simulink model "FOC_Controller"  (R2021a)
settings: Solver=FixedStepDiscrete  StartTime=0.0  StopTime=inf  FixedStep=4e-6  RelTol=1e-3
values from neighbouring files (symbols this model uses):
  FOC_bManualVdVq_C = Simulink.Parameter    [modeldata.m]
  FOC_iIdSP_C = Simulink.Parameter    [modeldata.m]
  FOC_kiPID_C = Simulink.Parameter    [modeldata.m]
  FOC_kpPID_C = Simulink.Parameter    [modeldata.m]
  FOC_uBusVoltage_C = Simulink.Parameter    [modeldata.m]
  FOC_uFindPosVd_C = Simulink.Parameter    [modeldata.m]
  FOC_uManualVd_C = Simulink.Parameter    [modeldata.m]
  FOC_uManualVq_C = Simulink.Parameter    [modeldata.m]
  Motor_bFindPosEnable_C = Simulink.Parameter    [modeldata.m]
  Motor_facTrq2Current_C = Simulink.Parameter    [modeldata.m]
  Motor_swtMode_C = Simulink.Parameter    [modeldata.m]
  Motor_tiFindPos_C = Simulink.Parameter    [modeldata.m]
  Motor_trqTorqueSetPoint_C = Simulink.Parameter    [modeldata.m]
  Position_degSetPoint_C = Simulink.Parameter    [modeldata.m]
  Position_kiPID_C = Simulink.Parameter    [modeldata.m]
  Position_kpPID_C = Simulink.Parameter    [modeldata.m]
  Position_nPIDMax_C = Simulink.Parameter    [modeldata.m]
  Speed_iPIDMax_C = Simulink.Parameter    [modeldata.m]
  Speed_kiPID_C = Simulink.Parameter    [modeldata.m]
  Speed_kpPID_C = Simulink.Parameter    [modeldata.m]
  Speed_nSetPoint_C = Simulink.Parameter    [modeldata.m]
  Speed_tiFilter_C = Simulink.Parameter    [modeldata.m]
libraries: simulink x11
(part 1 of 2)
settings Model: Creator=Administrator  LastModifiedBy=Administrator
settings SolverCC: AlgebraicLoopSolver=TrustRegion
settings DataIOCC: LimitDataPoints=on  ReturnWorkspaceOutputs=off
settings OptimizationCC: BlockReduction=off  DefaultParameterBehavior=Inlined  DefaultUnderspecifiedDataType=single  LifeSpan=1  EfficientTunableParamExpr=on
settings DebuggingCC: SignalInfNanChecking=warning  UnderspecifiedInitializationDetection=Classic  MergeDetectMultiDrivingBlocksExec=none  MultiTaskCondExecSysMsg=warning  MultiTaskRateTransMsg=warning  ParameterPrecisionLossMsg=none  SFUnexpectedBacktrackingDiag=warning  SFNoUnconditionalDefaultTransitionDiag=warning  SFExecutionAtInitializationDiag=none  SFMachineParentedDataDiag=warning  ArithmeticOperatorsInVariantConditions=warning
settings HardwareCC: ProdBitPerPointer=32  ProdBitPerSizeT=32  ProdBitPerPtrDiffT=32  ProdLargestAtomicInteger=Long  ProdLargestAtomicFloat=Double  ProdWordSize=32  ProdHWDeviceType=ARM Compatible->ARM Cortex
settings ModelReferenceCC: PropagateSignalLabelsOutOfModel=off
settings SFSimCC: SimUseLocalCustomCode=off  MATLABDynamicMemAlloc=off  CustomCodeUndefinedFunction=UseInterfaceOnly
settings RTWCC: SystemTargetFile=ert.tlc  GenCodeOnly=on  PackageName=AccPedal  TemplateMakefile=ert_default_tmf  GenerateReport=on  RTWVerbose=off  RTWUseLocalCustomCode=off  IncludeHyperlinkInReport=on  LaunchReport=on
settings CodeAppCC: IgnoreCustomStorageClasses=off  MaxIdLength=63  StateflowObjectComments=on
settings ERTTargetCC: TargetLangStandard=C99 (ISO)  MultiwordLength=2048  SupportNonFinite=off  ExtModeTransport=1  ExtModeMexFile=ext_serial_win32_comm  ERTCustomFileTemplate=example_file_process.tlc  ConvertIfToSwitch=off  SuppressUnreachableDefaultCases=off
settings ConfigComp: CovMetricSettings=dw  CovSaveCumulativeToWorkspaceVar=on  CovSaveSingleToWorkspaceVar=on  CovExternalEMLEnable=off  DVMaxProcessTime=600  DVMaxTestCaseSteps=500  DVTestSuiteOptimization=CombinedObjectives (Nonlinear Extended)  DVSaveReport=on
settings SimscapeCC: SimscapeNormalizeSystem=off

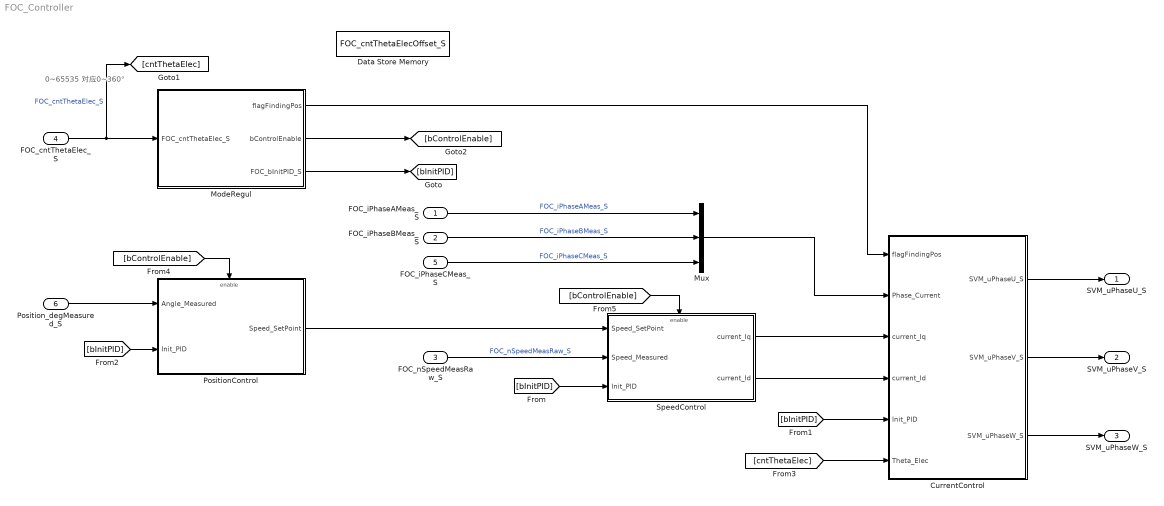
== system FOC_Controller ==
  note: 0~65535
      | 对应0~360°
  FOC_iPhaseAMeas_S : Inport  OutDataTypeStr=single
  FOC_iPhaseBMeas_S : Inport  Port=2  OutDataTypeStr=single
  FOC_nSpeedMeasRaw_S : Inport  Port=3
  FOC_cntThetaElec_S : Inport  Port=4
  FOC_iPhaseCMeas_S : Inport  Port=5  OutDataTypeStr=single
  Position_degMeasured_S : Inport  Port=6  OutDataTypeStr=single
  CurrentControl : Subsystem  TreatAsAtomicUnit=on  SystemSampleTime=200e-6  RTWFcnName=CurrentControl_Co  RTWFileName=CurrentControl
      settings: RTWSystemCode=Nonreusable function  RTWFcnNameOpts=User specified  RTWFileNameOpts=User specified
      settings: AttributesFormatString=|
      | ---------------------------------------
      | SampeTime = %<SystemSampleTime>
  Data Store Memory : DataStoreMemory  DataStoreName=FOC_cntThetaElecOffset_S  ReadBeforeWriteMsg=warning  WriteAfterWriteMsg=warning  WriteAfterReadMsg=warning  ShowAdditionalParam=off  StateMustResolveToSignalObject=on
  ModeRegul : Subsystem  TreatAsAtomicUnit=on  SystemSampleTime=0.05  RTWFcnName=ModeRegul_Co  RTWFileName=ModeRegul
      settings: RTWSystemCode=Nonreusable function  RTWFcnNameOpts=User specified  RTWFileNameOpts=User specified
      settings: AttributesFormatString=|
      | ---------------------------------------
      | SampeTime = %<SystemSampleTime>
  Mux : Mux  Inputs=3
  PositionControl : Subsystem  TreatAsAtomicUnit=on  SystemSampleTime=0.01  RTWFcnName=PositionControl_Co  RTWFileName=PositionControl
      settings: RTWSystemCode=Nonreusable function  RTWFcnNameOpts=User specified  RTWFileNameOpts=User specified
      settings: AttributesFormatString=|
      | ---------------------------------------
      | SampeTime = %<SystemSampleTime>
  SpeedControl : Subsystem  TreatAsAtomicUnit=on  SystemSampleTime=0.01  RTWFcnName=SpeedControl_Co  RTWFileName=SpeedControl
      settings: RTWSystemCode=Nonreusable function  RTWFcnNameOpts=User specified  RTWFileNameOpts=User specified
      settings: AttributesFormatString=|
      | ---------------------------------------
      | SampeTime = %<SystemSampleTime>
  SVM_uPhaseU_S : Outport  VectorParamsAs1DForOutWhenUnconnected=off
  SVM_uPhaseV_S : Outport  Port=2  VectorParamsAs1DForOutWhenUnconnected=off
  SVM_uPhaseW_S : Outport  Port=3  VectorParamsAs1DForOutWhenUnconnected=off
  wires:
  SpeedControl/1(current_Iq) -> CurrentControl/3(current_Iq)
  FOC_cntThetaElec_S/1 -> [cntThetaElec], ModeRegul/1(FOC_cntThetaElec_S)  "FOC_cntThetaElec_S"
  FOC_nSpeedMeasRaw_S/1 -> SpeedControl/2(Speed_Measured)  "FOC_nSpeedMeasRaw_S"
  Mux/1 -> CurrentControl/2(Phase_Current)
  [bInitPID] -> SpeedControl/3(Init_PID)
  FOC_iPhaseAMeas_S/1 -> Mux/1  "FOC_iPhaseAMeas_S"
  FOC_iPhaseBMeas_S/1 -> Mux/2  "FOC_iPhaseBMeas_S"
  FOC_iPhaseCMeas_S/1 -> Mux/3  "FOC_iPhaseCMeas_S"
  CurrentControl/1(SVM_uPhaseU_S) -> SVM_uPhaseU_S/1
  CurrentControl/3(SVM_uPhaseW_S) -> SVM_uPhaseW_S/1
  CurrentControl/2(SVM_uPhaseV_S) -> SVM_uPhaseV_S/1
  PositionControl/1(Speed_SetPoint) -> SpeedControl/1(Speed_SetPoint)
  [bInitPID] -> CurrentControl/5(Init_PID)
  Position_degMeasured_S/1 -> PositionControl/1(Angle_Measured)
  ModeRegul/3(FOC_bInitPID_S) -> [bInitPID]
  [bInitPID] -> PositionControl/2(Init_PID)
  [cntThetaElec] -> CurrentControl/6(Theta_Elec)
  ModeRegul/1(flagFindingPos) -> CurrentControl/1(flagFindingPos)
  ModeRegul/2(bControlEnable) -> [bControlEnable]
  [bControlEnable] -> PositionControl/Enable
  [bControlEnable] -> SpeedControl/Enable
  SpeedControl/2(current_Id) -> CurrentControl/4(current_Id)

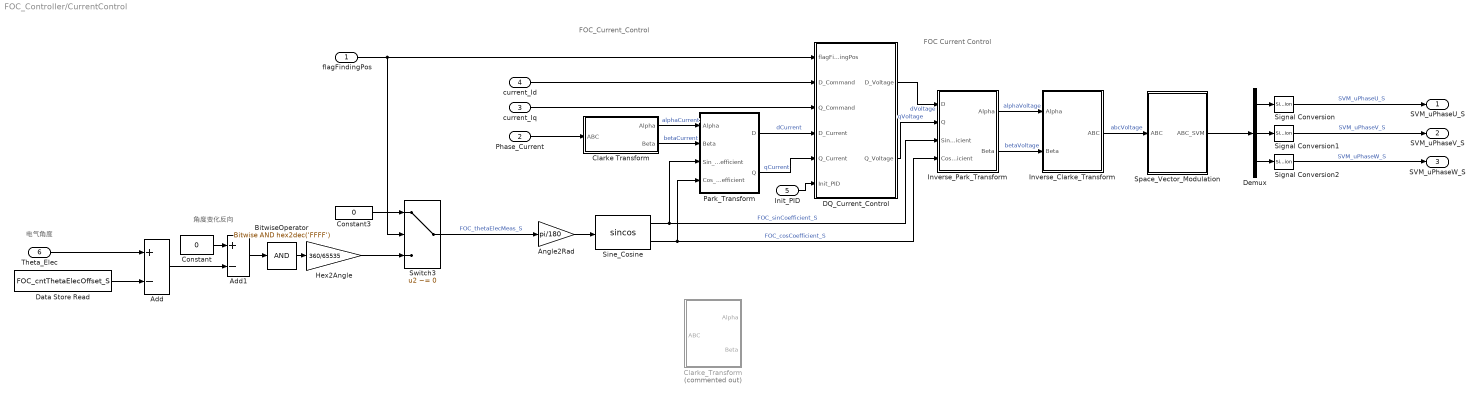
== system FOC_Controller/CurrentControl ==
  note: 角度变化反向
  note: 电气角度
  note: FOC Current Control
  note: FOC_Current_Control
  flagFindingPos : Inport
  Phase_Current : Inport  Port=2  OutDataTypeStr=single
  current_Iq : Inport  Port=3
  current_Id : Inport  Port=4
  Init_PID : Inport  Port=5  OutDataTypeStr=boolean
  Theta_Elec : Inport  Port=6  OutDataTypeStr=uint16
  Add : Sum  Inputs=+-  InputSameDT=on  OutDataTypeStr=Inherit: Same as first input
  Add1 : Sum  Inputs=+-  InputSameDT=on
  Angle2Rad : Gain  Gain=pi/180  OutDataTypeStr=Inherit: Inherit via back propagation  SaturateOnIntegerOverflow=on
  BitwiseOperator : simulink/Logic and Bit Operations/Bitwise Operator  logicop=AND  UseBitMask=on  BitMask=hex2dec('FFFF')  BitMaskRealWorld=Stored Integer
  Clarke Transform : Subsystem
      mask Display:
      | port_label('input',1,'ABC')
      | port_label('output',1,'\alpha','texmode', 'on')
      | port_label('output',2,'\beta','texmode', 'on')
  Clarke_Transform : Subsystem  Commented=on
      mask Display:
      | port_label('input',1,'ABC')
      | port_label('output',1,'\alpha','texmode', 'on')
      | port_label('output',2,'\beta','texmode', 'on')
  Constant : Constant  Value=0  OutDataTypeStr=uint16  SampleTime=-1
  Constant3 : Constant  Value=0  OutDataTypeStr=Inherit: Inherit via back propagation  SampleTime=-1
  DQ_Current_Control : Subsystem
  Data Store Read : DataStoreRead  DataStoreName=FOC_cntThetaElecOffset_S  IndexOptions=Index vector (dialog)  Indices=1  OutputSizes=1
  Demux : Demux  Outputs=3
  Hex2Angle : Gain  Gain=360/65535  OutDataTypeStr=Inherit: Inherit via back propagation  SaturateOnIntegerOverflow=on
  Inverse_Clarke_Transform : Subsystem  VariantControl=INVERSE_CLARKE_TRANSFORM
      mask Display:
      | port_label('input',1,'\alpha','texmode', 'on')
      | port_label('input',2,'\beta','texmode', 'on')
      | port_label('output',1,'ABC')
  Inverse_Park_Transform : Subsystem
      mask Display:
      | port_label('input',1,'D')
      | port_label('input',2,'Q')
      | port_label('input',3,'Sin')
      | port_label('input',4,'Cos')
      | port_label('output',1,'\alpha','texmode', 'on')
      | port_label('output',2,'\beta','texmode', 'on')
  Park_Transform : Subsystem
      mask Display:
      | port_label('input',1,'\alpha','texmode', 'on')
      | port_label('input',2,'\beta','texmode', 'on')
      | port_label('input',3,'Sin')
      | port_label('input',4,'Cos')
      | port_label('output',1,'D')
      | port_label('output',2,'Q')
  Signal Conversion : SignalConversion  OverrideOpt=off
  Signal Conversion1 : SignalConversion  OverrideOpt=off
  Signal Conversion2 : SignalConversion  OverrideOpt=off
  Sine_Cosine : Trigonometry  Operator=sincos
  Space_Vector_Modulation : Subsystem  VariantControl=SpaceVectorModulation_JB
      mask Display:
      | plot([0.000 0.020 0.041 0.061 0.082 0.102 0.122 0.143 0.163 0.184 0.204 0.224 0.245 0.265 0.286 0.306 0.327 0.347 0.367 0.388 0.408 0.429 0.449 0.469 0.490 0.510 0.531 0.551 0.571 0.592 0.612 0.633 0.653 0.673 0.694 0.714 0.735 0.755 0.776 0.796 0.816 0.837 0.857 0.878 0.898 0.918 0.939 0.959 0.980 1.000 ], ...
      |      [0.500 0.586 0.671 0.753 0.831 0.858 0.875 0.885 0.890 0.887 0.879 0.864 0.844 0.855 0.872 0.884 0.889 0.888 0.881 0.867 0.847 0.793 0.713 0.629 0.543 0.457 0.371 0.287 0.207 0.153 0.133 0.119 0.112 0.111 0.116 0.128 0.145 0.156 0.136 0.121 0.113 0.110 0.115 0.125 0.142 0.169 0.247 0.329 0.414 0.500 ])
  Switch3 : Switch  Criteria=u2 ~= 0  Threshold=1.5
  SVM_uPhaseU_S : Outport  VectorParamsAs1DForOutWhenUnconnected=off
  SVM_uPhaseV_S : Outport  Port=2  VectorParamsAs1DForOutWhenUnconnected=off
  SVM_uPhaseW_S : Outport  Port=3  VectorParamsAs1DForOutWhenUnconnected=off
  wires:
  Clarke Transform/2(Beta) -> Park_Transform/2(Beta)  "betaCurrent"
  Inverse_Clarke_Transform/1(ABC) -> Space_Vector_Modulation/1(ABC)  "abcVoltage"
  Phase_Current/1 -> Clarke Transform/1(ABC)
  Theta_Elec/1 -> Add/1
  Inverse_Park_Transform/2(Beta) -> Inverse_Clarke_Transform/2(Beta)  "betaVoltage"
  Sine_Cosine/1 -> Inverse_Park_Transform/3(Sin_Coefficient), Park_Transform/3(Sin_Coefficient)  "FOC_sinCoefficient_S"
  Space_Vector_Modulation/1(ABC_SVM) -> Demux/1
  Park_Transform/1(D) -> DQ_Current_Control/4(D_Current)  "dCurrent"
  Sine_Cosine/2 -> Inverse_Park_Transform/4(Cos_Coefficient), Park_Transform/4(Cos_Coefficient)  "FOC_cosCoefficient_S"
  Inverse_Park_Transform/1(Alpha) -> Inverse_Clarke_Transform/1(Alpha)  "alphaVoltage"
  Clarke Transform/1(Alpha) -> Park_Transform/1(Alpha)  "alphaCurrent"
  Park_Transform/2(Q) -> DQ_Current_Control/5(Q_Current)  "qCurrent"
  DQ_Current_Control/1(D_Voltage) -> Inverse_Park_Transform/1(D)  "dVoltage"
  DQ_Current_Control/2(Q_Voltage) -> Inverse_Park_Transform/2(Q)  "qVoltage"
  current_Iq/1 -> DQ_Current_Control/3(Q_Command)
  Init_PID/1 -> DQ_Current_Control/6(Init_PID)
  current_Id/1 -> DQ_Current_Control/2(D_Command)
  Constant3/1 -> Switch3/1
  Angle2Rad/1 -> Sine_Cosine/1
  Switch3/1 -> Angle2Rad/1  "FOC_thetaElecMeas_S"
  Hex2Angle/1 -> Switch3/3
  Data Store Read/1 -> Add/2
  BitwiseOperator/1 -> Hex2Angle/1
  Add1/1 -> BitwiseOperator/1
  Constant/1 -> Add1/1
  Add/1 -> Add1/2
  Signal Conversion/1 -> SVM_uPhaseU_S/1  "SVM_uPhaseU_S"
  Demux/2 -> Signal Conversion1/1
  Demux/3 -> Signal Conversion2/1
  Demux/1 -> Signal Conversion/1
  Signal Conversion1/1 -> SVM_uPhaseV_S/1  "SVM_uPhaseV_S"
  Signal Conversion2/1 -> SVM_uPhaseW_S/1  "SVM_uPhaseW_S"
  flagFindingPos/1 -> Switch3/2, DQ_Current_Control/1(flagFindingPos)

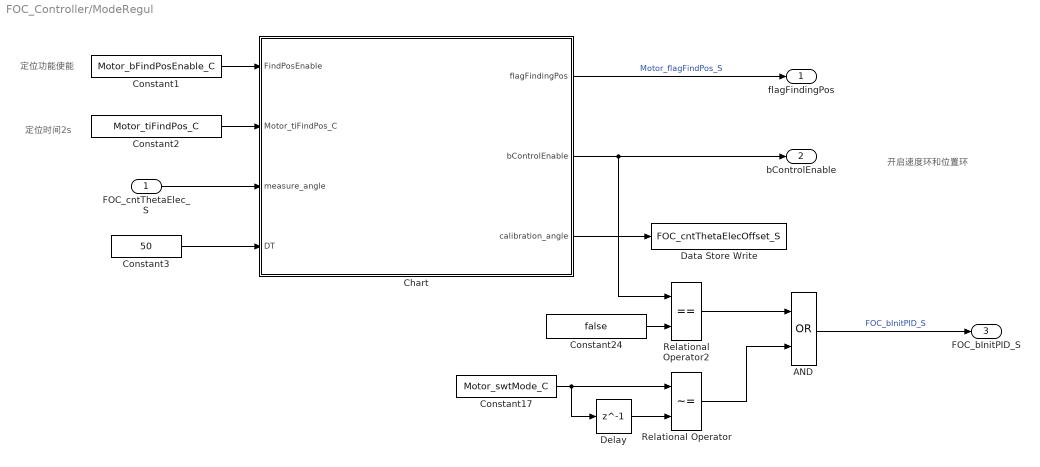
== system FOC_Controller/ModeRegul ==
  note: 开启速度环和位置环
  note: 定位功能使能
  note: 定位时间2s
  FOC_cntThetaElec_S : Inport
  AND : Logic  Operator=OR  AllPortsSameDT=off  OutDataTypeStr=boolean
  Chart : Stateflow chart  TreatAsAtomicUnit=on
  Constant1 : Constant  Value=Motor_bFindPosEnable_C  SampleTime=-1
  Constant17 : Constant  Value=Motor_swtMode_C  SampleTime=-1
  Constant2 : Constant  Value=Motor_tiFindPos_C  SampleTime=-1
  Constant24 : Constant  Value=false  OutDataTypeStr=Inherit: Inherit via back propagation  SampleTime=-1
  Constant3 : Constant  Value=50  OutDataTypeStr=Inherit: Inherit via back propagation  SampleTime=-1
  Data Store Write : DataStoreWrite  DataStoreName=FOC_cntThetaElecOffset_S  IndexOptions=Index vector (dialog)  Indices=1  OutputSizes=1
  Delay : Delay  DelayLength=1  InitialCondition=0
  Relational Operator : RelationalOperator  Operator=~=  OutDataTypeStr=boolean  RndMeth=Simplest  InputSameDT=on
  Relational Operator2 : RelationalOperator  Operator===  OutDataTypeStr=boolean  RndMeth=Simplest  InputSameDT=on
  flagFindingPos : Outport  VectorParamsAs1DForOutWhenUnconnected=off
  bControlEnable : Outport  Port=2  VectorParamsAs1DForOutWhenUnconnected=off
  FOC_bInitPID_S : Outport  Port=3  VectorParamsAs1DForOutWhenUnconnected=off
  wires:
  Constant3/1 -> Chart/4(DT)
  Constant1/1 -> Chart/1(FindPosEnable)
  Constant2/1 -> Chart/2(Motor_tiFindPos_C)
  FOC_cntThetaElec_S/1 -> Chart/3(measure_angle)
  Chart/1(flagFindingPos) -> flagFindingPos/1  "Motor_flagFindPos_S"
  Chart/2(bControlEnable) -> Relational Operator2/1, bControlEnable/1
  Chart/3(calibration_angle) -> Data Store Write/1
  Delay/1 -> Relational Operator/2
  Constant17/1 -> Delay/1, Relational Operator/1
  Constant24/1 -> Relational Operator2/2
  Relational Operator2/1 -> AND/1
  AND/1 -> FOC_bInitPID_S/1  "FOC_bInitPID_S"
  Relational Operator/1 -> AND/2

== system FOC_Controller/PositionControl ==
  Angle_Measured : Inport  OutDataTypeStr=single
  Init_PID : Inport  Port=2  OutDataTypeStr=boolean
  Enable : EnablePort
  Constant8 : Constant  Value=Position_degSetPoint_C  SampleTime=-1
  Position_Control : Subsystem
      mask Display:
      | port_label('input',1,'SetPoint','texmode', 'on')
      | port_label('input',2,'Measured','texmode', 'on')
      | port_label('input',3,'Kp')
      | port_label('input',4,'Ki')
      | port_label('input',5,'Init')
      | port_label('input',6,'Max')
      | port_label('output',1,'Out')
  ki_0.12 : Constant  Value=Position_kiPID_C  SampleTime=-1
  kp_0.0015 : Constant  Value=Position_kpPID_C  SampleTime=-1
  paramPositionControlSatCurrent_4 : Constant  Value=Position_nPIDMax_C  OutDataTypeStr=Inherit: Inherit via back propagation  SampleTime=-1
  Speed_SetPoint : Outport  VectorParamsAs1DForOutWhenUnconnected=off
  wires:
  ki_0.12/1 -> Position_Control/4(Current_Ki)
  kp_0.0015/1 -> Position_Control/3(Current_Kp)
  Angle_Measured/1 -> Position_Control/2(Current_Measured)  "Position_degMeasured_S"
  Init_PID/1 -> Position_Control/5(Init_PID)
  paramPositionControlSatCurrent_4/1 -> Position_Control/6(PID_max)
  Position_Control/1(Voltage_Vd) -> Speed_SetPoint/1
  Constant8/1 -> Position_Control/1(Current_Command)

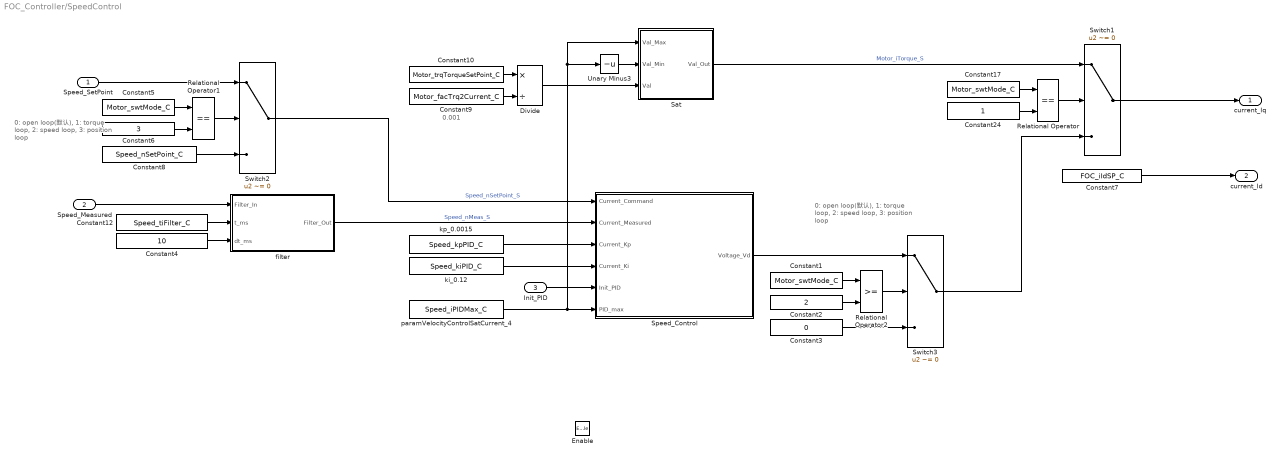
== system FOC_Controller/SpeedControl ==
  note: 0.001
  note: 0: open loop(默认),
      | 1: torque loop,
      | 2: speed loop,
      | 3: position loop
  note: 0: open loop(默认),
      | 1: torque loop,
      | 2: speed loop,
      | 3: position loop
  Speed_SetPoint : Inport  OutDataTypeStr=single
  Speed_Measured : Inport  Port=2  OutDataTypeStr=single
  Init_PID : Inport  Port=3  OutDataTypeStr=boolean
  Enable : EnablePort
  Constant1 : Constant  Value=Motor_swtMode_C  SampleTime=-1
  Constant10 : Constant  Value=Motor_trqTorqueSetPoint_C  SampleTime=-1
  Constant12 : Constant  Value=Speed_tiFilter_C  SampleTime=-1
  Constant17 : Constant  Value=Motor_swtMode_C  SampleTime=-1
  Constant2 : Constant  Value=2  OutDataTypeStr=Inherit: Inherit via back propagation  SampleTime=-1
  Constant24 : Constant  OutDataTypeStr=Inherit: Inherit via back propagation  SampleTime=-1
  Constant3 : Constant  Value=0  OutDataTypeStr=Inherit: Inherit via back propagation  SampleTime=-1
  Constant4 : Constant  Value=10  OutDataTypeStr=Inherit: Inherit via back propagation  SampleTime=-1
  Constant5 : Constant  Value=Motor_swtMode_C  SampleTime=-1
  Constant6 : Constant  Value=3  OutDataTypeStr=Inherit: Inherit via back propagation  SampleTime=-1
  Constant7 : Constant  Value=FOC_iIdSP_C  OutDataTypeStr=Inherit: Inherit via back propagation  SampleTime=-1
  Constant8 : Constant  Value=Speed_nSetPoint_C  SampleTime=-1
  Constant9 : Constant  Value=Motor_facTrq2Current_C  SampleTime=-1
  Divide : Product  Inputs=*/  OutDataTypeStr=Inherit: Inherit via back propagation  RndMeth=Zero  SaturateOnIntegerOverflow=on
  Relational Operator : RelationalOperator  Operator===  OutDataTypeStr=boolean  RndMeth=Simplest  InputSameDT=on
  Relational Operator1 : RelationalOperator  Operator===  OutDataTypeStr=boolean  RndMeth=Simplest  InputSameDT=on
  Relational Operator2 : RelationalOperator  OutDataTypeStr=boolean  RndMeth=Simplest  InputSameDT=on
  Sat : Subsystem
      mask Display:
      | port_label('input',1,'ValMax','texmode', 'on')
      | port_label('input',2,'ValMin','texmode', 'on')
      | port_label('input',3,'Val')
      | port_label('output',1,'Val_Out')
  Speed_Control : Subsystem
      mask Display:
      | port_label('input',1,'SetPoint','texmode', 'on')
      | port_label('input',2,'Measured','texmode', 'on')
      | port_label('input',3,'Kp')
      | port_label('input',4,'Ki')
      | port_label('input',5,'Init')
      | port_label('input',6,'Max')
      | port_label('output',1,'Out')
  Switch1 : Switch  Criteria=u2 ~= 0  Threshold=1.5
  Switch2 : Switch  Criteria=u2 ~= 0  Threshold=1.5
  Switch3 : Switch  Criteria=u2 ~= 0  Threshold=1.5
  Unary Minus3 : UnaryMinus
  filter : Subsystem  AncestorBlock=XidoorLib/Software/filter  TreatAsAtomicUnit=on  RTWFcnName=lib_filter  RTWFileName=CurrentControl  mask(PT1_S16){}
      mask help:
      | PT1滤波：用于消除信号干扰，平滑过渡阶跃等；
      |
      | In1（PT_fac）: factor，滤波系数（0~100%），默认设置为50；
      | In2（int8/uint8/int16/uint16/int32/uint32）: input；
      |
      | Out1: result
      settings: RTWFcnNameOpts=User specified  RTWFileNameOpts=User specified
      mask Display:
      | %image('.\Pic\PT1Control.jpg')
      | set_param(gcb, 'BackgroundColor', '[0.454902, 0.901961, 0.737255]');
      | disp('{\bffilter}','texmode','on');
  ki_0.12 : Constant  Value=Speed_kiPID_C  SampleTime=-1
  kp_0.0015 : Constant  Value=Speed_kpPID_C  SampleTime=-1
  paramVelocityControlSatCurrent_4 : Constant  Value=Speed_iPIDMax_C  OutDataTypeStr=Inherit: Inherit via back propagation  SampleTime=-1
  current_Iq : Outport  VectorParamsAs1DForOutWhenUnconnected=off
  current_Id : Outport  Port=2  VectorParamsAs1DForOutWhenUnconnected=off
  wires:
  Speed_Control/1(Voltage_Vd) -> Switch3/1
  ki_0.12/1 -> Speed_Control/4(Current_Ki)
  kp_0.0015/1 -> Speed_Control/3(Current_Kp)
  filter/1(Filter_Out) -> Speed_Control/2(Current_Measured)  "Speed_nMeas_S"
  Init_PID/1 -> Speed_Control/5(Init_PID)
  Unary Minus3/1 -> Sat/2(Val_Min)
  Relational Operator/1 -> Switch1/2
  Constant24/1 -> Relational Operator/2
  paramVelocityControlSatCurrent_4/1 -> Speed_Control/6(PID_max), Sat/1(Val_Max), Unary Minus3/1
  Constant9/1 -> Divide/2
  Sat/1(Val_Out) -> Switch1/1  "Motor_iTorque_S"
  Constant10/1 -> Divide/1
  Divide/1 -> Sat/3(Val)
  Constant17/1 -> Relational Operator/1
  Switch1/1 -> current_Iq/1
  Constant8/1 -> Switch2/3
  Constant12/1 -> filter/2(t_ms)
  Speed_Measured/1 -> filter/1(Filter_In)
  Constant4/1 -> filter/3(dt_ms)
  Constant5/1 -> Relational Operator1/1
  Constant6/1 -> Relational Operator1/2
  Relational Operator1/1 -> Switch2/2
  Switch2/1 -> Speed_Control/1(Current_Command)  "Speed_nSetPoint_S"
  Speed_SetPoint/1 -> Switch2/1
  Constant1/1 -> Relational Operator2/1
  Relational Operator2/1 -> Switch3/2
  Constant2/1 -> Relational Operator2/2
  Switch3/1 -> Switch1/3
  Constant3/1 -> Switch3/3
  Constant7/1 -> current_Id/1

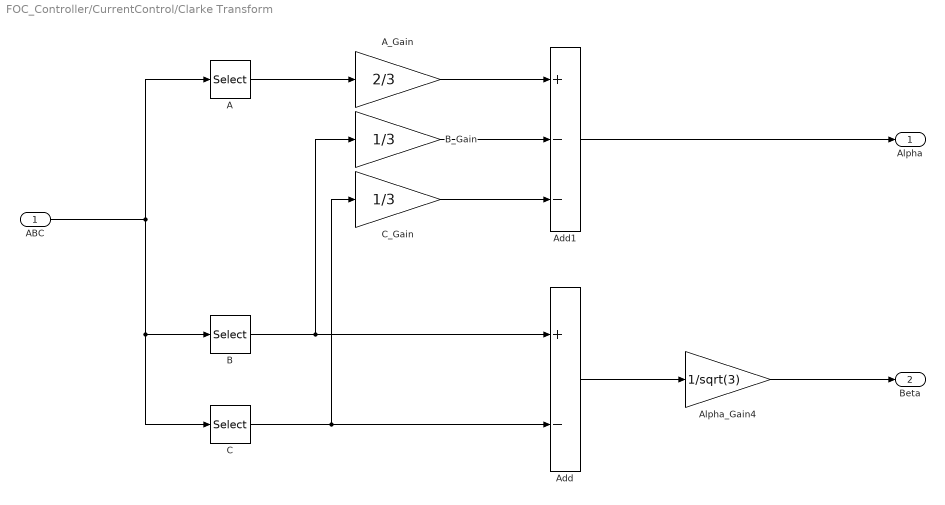
== system FOC_Controller/CurrentControl/Clarke Transform ==
  ABC : Inport
  A : Selector  IndexMode=Zero-based  InputPortWidth=3  IndexOptions=Index vector (dialog)  Indices=0  OutputSizes=1
  A_Gain : Gain  Gain=2/3
  Add : Sum  Inputs=+-  OutDataTypeStr=Inherit: Same as first input
  Add1 : Sum  Inputs=+--  OutDataTypeStr=Inherit: Same as first input
  Alpha_Gain4 : Gain  Gain=1/sqrt(3)
  B : Selector  IndexMode=Zero-based  InputPortWidth=3  IndexOptions=Index vector (dialog)  Indices=1  OutputSizes=1
  B_Gain : Gain  Gain=1/3
  C : Selector  IndexMode=Zero-based  InputPortWidth=3  IndexOptions=Index vector (dialog)  Indices=2  OutputSizes=1
  C_Gain : Gain  Gain=1/3
  Alpha : Outport  VectorParamsAs1DForOutWhenUnconnected=off
  Beta : Outport  Port=2  VectorParamsAs1DForOutWhenUnconnected=off
  wires:
  B/1 -> B_Gain/1, Add/1
  ABC/1 -> A/1, C/1, B/1
  Add/1 -> Alpha_Gain4/1
  A/1 -> A_Gain/1
  A_Gain/1 -> Add1/1
  B_Gain/1 -> Add1/2
  C/1 -> C_Gain/1, Add/2
  C_Gain/1 -> Add1/3
  Add1/1 -> Alpha/1
  Alpha_Gain4/1 -> Beta/1

== system FOC_Controller/CurrentControl/Clarke_Transform ==
  note: Clarke Transform
  note: Converts balanced three-phase quantities into balanced two-phase quantities.
      | The A and B phases are converted to the direct axis (alpha) component and the quadrature axis (beta) component.
      | The alpha and beta components are still dependent on time and speed.
  ABC : Inport
  A : Selector  IndexMode=Zero-based  InputPortWidth=2  IndexOptions=Index vector (dialog)  Indices=0  OutputSizes=1
  Add : Sum  OutDataTypeStr=Inherit: Same as first input
  Alpha_Gain : Gain  Gain=1/sqrt(3)
  B : Selector  IndexMode=Zero-based  InputPortWidth=2  IndexOptions=Index vector (dialog)  Indices=1  OutputSizes=1
  Beta_Gain : Gain  Gain=2/sqrt(3)
  Alpha : Outport  VectorParamsAs1DForOutWhenUnconnected=off
  Beta : Outport  Port=2  VectorParamsAs1DForOutWhenUnconnected=off
  wires:
  Add/1 -> Beta/1
  B/1 -> Beta_Gain/1
  Beta_Gain/1 -> Add/2
  ABC/1 -> A/1, B/1
  Alpha_Gain/1 -> Add/1
  A/1 -> Alpha_Gain/1, Alpha/1

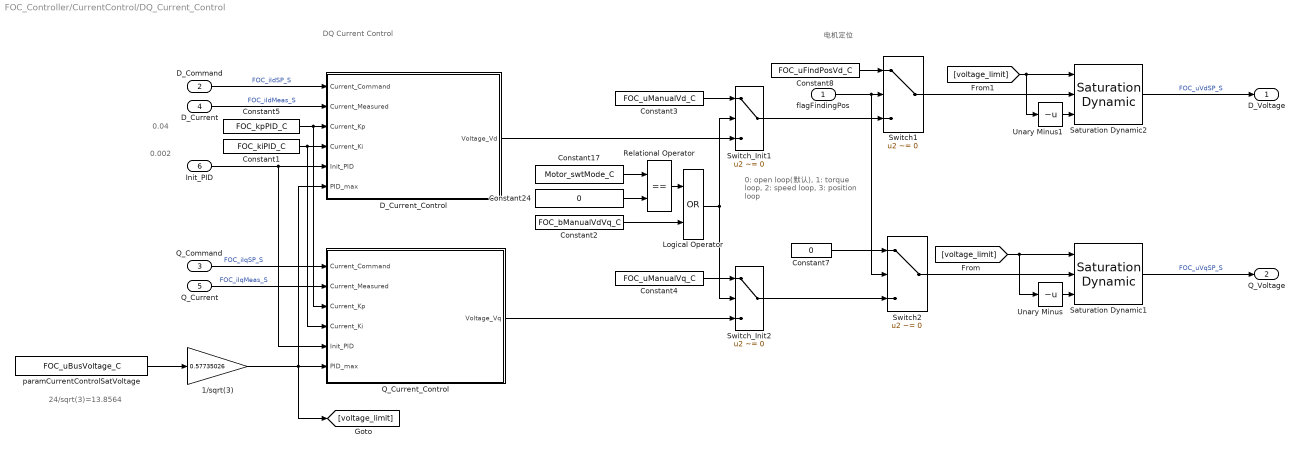
== system FOC_Controller/CurrentControl/DQ_Current_Control ==
  note: 电机定位
  note: 0.002
  note: 0.04
  note: DQ Current Control
  note: 24/sqrt(3)=13.8564
  note: 0: open loop(默认),
      | 1: torque loop,
      | 2: speed loop,
      | 3: position loop
  flagFindingPos : Inport
  D_Command : Inport  Port=2
  Q_Command : Inport  Port=3
  D_Current : Inport  Port=4
  Q_Current : Inport  Port=5
  Init_PID : Inport  Port=6  OutDataTypeStr=boolean
  1/sqrt(3) : Gain  Gain=0.57735026
  Constant1 : Constant  Value=FOC_kiPID_C  OutDataTypeStr=Inherit: Inherit via back propagation  SampleTime=-1
  Constant17 : Constant  Value=Motor_swtMode_C  SampleTime=-1
  Constant2 : Constant  Value=FOC_bManualVdVq_C  OutDataTypeStr=Inherit: Inherit via back propagation  SampleTime=-1
  Constant24 : Constant  Value=0  OutDataTypeStr=Inherit: Inherit via back propagation  SampleTime=-1
  Constant3 : Constant  Value=FOC_uManualVd_C  OutDataTypeStr=Inherit: Inherit via back propagation  SampleTime=-1
  Constant4 : Constant  Value=FOC_uManualVq_C  OutDataTypeStr=Inherit: Inherit via back propagation  SampleTime=-1
  Constant5 : Constant  Value=FOC_kpPID_C  OutDataTypeStr=Inherit: Inherit via back propagation  SampleTime=-1
  Constant7 : Constant  Value=0  OutDataTypeStr=Inherit: Inherit via back propagation  SampleTime=-1
  Constant8 : Constant  Value=FOC_uFindPosVd_C  OutDataTypeStr=Inherit: Inherit via back propagation  SampleTime=-1
  D_Current_Control : Subsystem
      mask Display:
      | port_label('input',1,'SetPoint','texmode', 'on')
      | port_label('input',2,'Measured','texmode', 'on')
      | port_label('input',3,'Kp')
      | port_label('input',4,'Ki')
      | port_label('input',5,'Init')
      | port_label('input',6,'Max')
      | port_label('output',1,'Out')
  Logical Operator : Logic  Operator=OR  AllPortsSameDT=off  OutDataTypeStr=boolean
  Q_Current_Control : Subsystem
      mask Display:
      | port_label('input',1,'SetPoint','texmode', 'on')
      | port_label('input',2,'Measured','texmode', 'on')
      | port_label('input',3,'Kp')
      | port_label('input',4,'Ki')
      | port_label('input',5,'Init')
      | port_label('input',6,'Max')
      | port_label('output',1,'Out')
  Relational Operator : RelationalOperator  Operator===  OutDataTypeStr=boolean  RndMeth=Simplest  InputSameDT=on
  Saturation Dynamic1 : simulink/Discontinuities/Saturation Dynamic  OutMin=[]  OutMax=[]  OutDataTypeStr=Inherit: Same as second input  OutDataType=fixdt(1, 16)  OutScaling=2^-10  DoSatur=off
  Saturation Dynamic2 : simulink/Discontinuities/Saturation Dynamic  OutMin=[]  OutMax=[]  OutDataTypeStr=Inherit: Same as second input  OutDataType=fixdt(1, 16)  OutScaling=2^-10  DoSatur=off
  Switch1 : Switch  Criteria=u2 ~= 0  Threshold=1.5
  Switch2 : Switch  Criteria=u2 ~= 0  Threshold=1.5
  Switch_Init1 : Switch  Criteria=u2 ~= 0  OutDataTypeStr=Inherit: Inherit via back propagation  InputSameDT=on
  Switch_Init2 : Switch  Criteria=u2 ~= 0  OutDataTypeStr=Inherit: Inherit via back propagation  InputSameDT=on
  Unary Minus : UnaryMinus
  Unary Minus1 : UnaryMinus
  paramCurrentControlSatVoltage : Constant  Value=FOC_uBusVoltage_C  SampleTime=-1
  D_Voltage : Outport  VectorParamsAs1DForOutWhenUnconnected=off
  Q_Voltage : Outport  Port=2  VectorParamsAs1DForOutWhenUnconnected=off
  wires:
  Q_Current_Control/1(Voltage_Vq) -> Switch_Init2/3
  Saturation Dynamic2/1 -> D_Voltage/1  "FOC_uVdSP_S"
  Q_Command/1 -> Q_Current_Control/1(Current_Command)  "FOC_iIqSP_S"
  Q_Current/1 -> Q_Current_Control/2(Current_Measured)  "FOC_iIqMeas_S"
  D_Current/1 -> D_Current_Control/2(Current_Measured)  "FOC_iIdMeas_S"
  Constant5/1 -> Q_Current_Control/3(Current_Kp), D_Current_Control/3(Current_Kp)
  Constant1/1 -> Q_Current_Control/4(Current_Ki), D_Current_Control/4(Current_Ki)
  Init_PID/1 -> Q_Current_Control/5(Init_PID), D_Current_Control/5(Init_PID)
  1/sqrt(3)/1 -> [voltage_limit], D_Current_Control/6(PID_max), Q_Current_Control/6(PID_max)
  D_Command/1 -> D_Current_Control/1(Current_Command)  "FOC_iIdSP_S"
  D_Current_Control/1(Voltage_Vd) -> Switch_Init1/3
  Constant3/1 -> Switch_Init1/1
  Constant4/1 -> Switch_Init2/1
  Saturation Dynamic1/1 -> Q_Voltage/1  "FOC_uVqSP_S"
  Constant24/1 -> Relational Operator/2
  Constant17/1 -> Relational Operator/1
  Relational Operator/1 -> Logical Operator/1
  Constant2/1 -> Logical Operator/2
  Logical Operator/1 -> Switch_Init1/2, Switch_Init2/2
  paramCurrentControlSatVoltage/1 -> 1/sqrt(3)/1
  Constant8/1 -> Switch1/1
  Constant7/1 -> Switch2/1
  Switch_Init1/1 -> Switch1/3
  Switch_Init2/1 -> Switch2/3
  flagFindingPos/1 -> Switch2/2, Switch1/2
  Switch1/1 -> Saturation Dynamic2/2
  Switch2/1 -> Saturation Dynamic1/2
  Unary Minus/1 -> Saturation Dynamic1/3
  [voltage_limit] -> Unary Minus/1, Saturation Dynamic1/1
  [voltage_limit] -> Unary Minus1/1, Saturation Dynamic2/1
  Unary Minus1/1 -> Saturation Dynamic2/3

== system FOC_Controller/CurrentControl/Inverse_Clarke_Transform ==
  note: InvVds
  note: Inverse Clarke Transform
  note: Converts direct axis (alpha) component and the quadrature axis (beta) component to balanced three-phase quantities
      | The alpha and beta components are dependent on time and speed.
  note: InvVqs
  Alpha : Inport
  Beta : Inport  Port=2
  Add : Sum  Inputs=-+  OutDataTypeStr=Inherit: Same as first input
  Add1 : Sum  Inputs=--  OutDataTypeStr=Inherit: Same as first input
  Gain : Gain  Gain=1/2
  Gain1 : Gain  Gain=sqrt(3)/2
  Mux : Mux  Inputs=3
  ABC : Outport  VectorParamsAs1DForOutWhenUnconnected=off
  wires:
  Gain/1 -> Add1/1, Add/1
  Gain1/1 -> Add1/2, Add/2
  Add/1 -> Mux/2  "FOC_uPhaseVVolt_S"
  Add1/1 -> Mux/3  "FOC_uPhaseWVolt_S"
  Beta/1 -> Gain1/1
  Alpha/1 -> Mux/1, Gain/1  "FOC_uPhaseUVolt_S"
  Mux/1 -> ABC/1

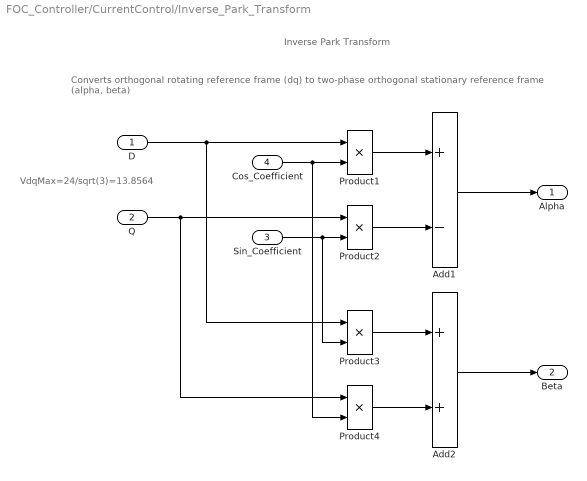
== system FOC_Controller/CurrentControl/Inverse_Park_Transform ==
  note: Inverse Park Transform
  note: Converts orthogonal rotating reference frame (dq) to two-phase orthogonal stationary reference frame (alpha, beta)
  note: VdqMax=24/sqrt(3)=13.8564
  D : Inport
  Q : Inport  Port=2
  Sin_Coefficient : Inport  Port=3
  Cos_Coefficient : Inport  Port=4
  Add1 : Sum  Inputs=+-  OutDataTypeStr=Inherit: Same as first input
  Add2 : Sum  OutDataTypeStr=Inherit: Same as first input
  Product{1..4} (4 alike) : Product  RndMeth=Simplest
  Alpha : Outport  VectorParamsAs1DForOutWhenUnconnected=off
  Beta : Outport  Port=2  VectorParamsAs1DForOutWhenUnconnected=off
  wires:
  Add2/1 -> Beta/1
  Add1/1 -> Alpha/1
  Product3/1 -> Add2/1
  Product4/1 -> Add2/2
  Product1/1 -> Add1/1
  Product2/1 -> Add1/2
  Cos_Coefficient/1 -> Product4/2, Product1/2
  D/1 -> Product3/1, Product1/1
  Q/1 -> Product2/1, Product4/1
  Sin_Coefficient/1 -> Product3/2, Product2/2

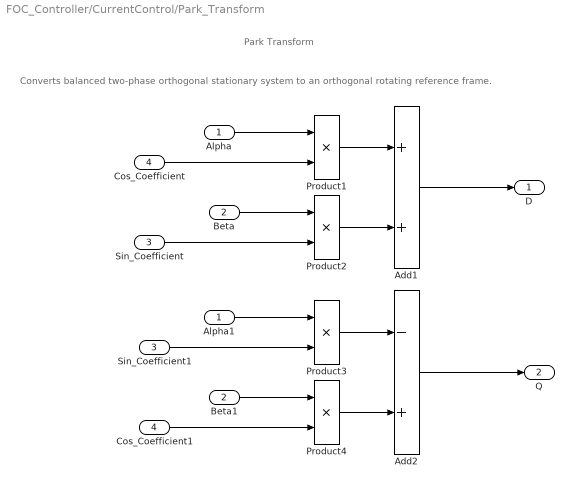
== system FOC_Controller/CurrentControl/Park_Transform ==
  note: Park Transform
  note: Converts balanced two-phase orthogonal stationary system to an orthogonal rotating reference frame.
  Alpha : Inport
  Beta : Inport  Port=2
  Sin_Coefficient : Inport  Port=3
  Cos_Coefficient : Inport  Port=4
  Add1 : Sum  OutDataTypeStr=Inherit: Same as first input
  Add2 : Sum  Inputs=-+  OutDataTypeStr=Inherit: Same as first input
  Alpha1 : InportShadow
  Beta1 : InportShadow  Port=2
  Cos_Coefficient1 : InportShadow  Port=4
  Product{1..4} (4 alike) : Product  RndMeth=Simplest
  Sin_Coefficient1 : InportShadow  Port=3
  D : Outport  VectorParamsAs1DForOutWhenUnconnected=off
  Q : Outport  Port=2  VectorParamsAs1DForOutWhenUnconnected=off
  wires:
  Product3/1 -> Add2/1
  Product4/1 -> Add2/2
  Product1/1 -> Add1/1
  Product2/1 -> Add1/2
  Alpha1/1 -> Product3/1
  Sin_Coefficient1/1 -> Product3/2
  Cos_Coefficient1/1 -> Product4/2
  Beta1/1 -> Product4/1
  Alpha/1 -> Product1/1
  Cos_Coefficient/1 -> Product1/2
  Beta/1 -> Product2/1
  Sin_Coefficient/1 -> Product2/2
  Add1/1 -> D/1
  Add2/1 -> Q/1

== system FOC_Controller/CurrentControl/Space_Vector_Modulation ==
  note: Space Vector Modulation
  ABC : Inport
  Add : Sum
  Add1 : Sum  Inputs=+-
  Gain : Gain  Gain=0.5  OutDataTypeStr=Inherit: Same as input
  Max : MinMax  Function=max
  Min : MinMax
  ABC_SVM : Outport  VectorParamsAs1DForOutWhenUnconnected=off
  wires:
  Add/1 -> Gain/1
  Max/1 -> Add/1
  Min/1 -> Add/2
  Gain/1 -> Add1/2
  ABC/1 -> Min/1, Max/1, Add1/1
  Add1/1 -> ABC_SVM/1

== system FOC_Controller/PositionControl/Position_Control ==
  note: D Current Control
  Current_Command : Inport
  Current_Measured : Inport  Port=2
  Current_Kp : Inport  Port=3
  Current_Ki : Inport  Port=4
  Init_PID : Inport  Port=5  OutDataTypeStr=boolean
  PID_max : Inport  Port=6
  Constant5 : Constant  Value=0  OutDataTypeStr=Inherit: Inherit via back propagation  SampleTime=-1
  Error : Sum  Inputs=+-
  PID : Subsystem  TreatAsAtomicUnit=on
  Voltage_Vd : Outport  VectorParamsAs1DForOutWhenUnconnected=off
  wires:
  Error/1 -> PID/1(Differ)  "currentControlError"
  Current_Command/1 -> Error/1
  Current_Measured/1 -> Error/2  "current"
  Current_Kp/1 -> PID/2(Kp)
  Init_PID/1 -> PID/5(Init)
  Current_Ki/1 -> PID/3(Ki)
  Constant5/1 -> PID/4(Kd)
  PID_max/1 -> PID/6(Sat_value)
  PID/1(PID_Out) -> Voltage_Vd/1

== system FOC_Controller/SpeedControl/Sat ==
  Val_Max : Inport
  Val_Min : Inport  Port=2
  Val : Inport  Port=3
  Relational Operator : RelationalOperator  Operator=>  OutDataTypeStr=boolean  RndMeth=Nearest  InputSameDT=on
  Relational Operator1 : RelationalOperator  Operator=<=  OutDataTypeStr=boolean  RndMeth=Nearest  InputSameDT=on
  Switch_Inf : Switch  Criteria=u2 > Threshold
  Switch_Sup : Switch  Criteria=u2 > Threshold
  Val_Out : Outport  VectorParamsAs1DForOutWhenUnconnected=off
  wires:
  Switch_Inf/1 -> Val_Out/1
  Switch_Sup/1 -> Relational Operator/1, Switch_Inf/1
  Relational Operator1/1 -> Switch_Sup/2
  Val_Max/1 -> Switch_Sup/1, Relational Operator1/1
  Val/1 -> Switch_Sup/3, Relational Operator1/2
  Val_Min/1 -> Switch_Inf/3, Relational Operator/2
  Relational Operator/1 -> Switch_Inf/2

== system FOC_Controller/SpeedControl/Speed_Control ==
  note: D Current Control
  note: 24/sqrt(3)=13.8564
  Current_Command : Inport
  Current_Measured : Inport  Port=2
  Current_Kp : Inport  Port=3
  Current_Ki : Inport  Port=4
  Init_PID : Inport  Port=5  OutDataTypeStr=boolean
  PID_max : Inport  Port=6
  Constant5 : Constant  Value=0  OutDataTypeStr=Inherit: Inherit via back propagation  SampleTime=-1
  Error : Sum  Inputs=+-
  PID : Subsystem  TreatAsAtomicUnit=on
  Voltage_Vd : Outport  VectorParamsAs1DForOutWhenUnconnected=off
  wires:
  Error/1 -> PID/1(Differ)  "currentControlError"
  Current_Command/1 -> Error/1
  Current_Measured/1 -> Error/2  "current"
  Current_Kp/1 -> PID/2(Kp)
  Init_PID/1 -> PID/5(Init)
  Current_Ki/1 -> PID/3(Ki)
  Constant5/1 -> PID/4(Kd)
  PID_max/1 -> PID/6(Sat_value)
  PID/1(PID_Out) -> Voltage_Vd/1

== system FOC_Controller/SpeedControl/filter ==
  note: Yn=a*Xn+(1-a)Yn-1
  Filter_In : Inport
  t_ms : Inport  Port=2
  dt_ms : Inport  Port=3
  Add : Sum  InputSameDT=on  OutDataTypeStr=Inherit: Inherit via back propagation  SaturateOnIntegerOverflow=on
  Add1 : Sum  Inputs=+-  InputSameDT=on
  Add2 : Sum  InputSameDT=on
  Constant : Constant  OutDataTypeStr=Inherit: Inherit via back propagation  SampleTime=-1
  Delay : Delay  DelayLength=1  InitialCondition=0
  Product : Product  SaturateOnIntegerOverflow=on  OutDataTypeStr=Inherit: Same as first input
  Product1 : Product  Inputs=*/  OutDataTypeStr=Inherit: Inherit via back propagation  SaturateOnIntegerOverflow=on
  Product2 : Product  SaturateOnIntegerOverflow=on  OutDataTypeStr=Inherit: Same as first input
  Filter_Out : Outport  VectorParamsAs1DForOutWhenUnconnected=off
  wires:
  Delay/1 -> Product/1  "Yn-1"
  Add2/1 -> Product1/2
  Product2/1 -> Add/2
  Constant/1 -> Add1/1
  t_ms/1 -> Add2/1
  dt_ms/1 -> Product1/1, Add2/2
  Add/1 -> Delay/1, Filter_Out/1  "Yn"
  Product/1 -> Add/1
  Product1/1 -> Add1/2, Product2/1  "a"
  Add1/1 -> Product/2
  Filter_In/1 -> Product2/2  "Xn"

== system FOC_Controller/CurrentControl/DQ_Current_Control/D_Current_Control ==
  note: D Current Control
  note: 24/sqrt(3)=13.8564
  Current_Command : Inport
  Current_Measured : Inport  Port=2
  Current_Kp : Inport  Port=3
  Current_Ki : Inport  Port=4
  Init_PID : Inport  Port=5  OutDataTypeStr=boolean
  PID_max : Inport  Port=6
  Constant5 : Constant  Value=0  OutDataTypeStr=Inherit: Inherit via back propagation  SampleTime=-1
  Error : Sum  Inputs=+-
  PID : Subsystem  TreatAsAtomicUnit=on
  Voltage_Vd : Outport  VectorParamsAs1DForOutWhenUnconnected=off
  wires:
  Error/1 -> PID/1(Differ)  "currentControlError"
  Current_Command/1 -> Error/1
  Current_Measured/1 -> Error/2  "current"
  Current_Kp/1 -> PID/2(Kp)
  Init_PID/1 -> PID/5(Init)
  Current_Ki/1 -> PID/3(Ki)
  Constant5/1 -> PID/4(Kd)
  PID_max/1 -> PID/6(Sat_value)
  PID/1(PID_Out) -> Voltage_Vd/1

== system FOC_Controller/CurrentControl/DQ_Current_Control/Q_Current_Control ==
  note: 24/sqrt(3)=13.8564
  note: Q Current Control
  Current_Command : Inport
  Current_Measured : Inport  Port=2
  Current_Kp : Inport  Port=3
  Current_Ki : Inport  Port=4
  Init_PID : Inport  Port=5  OutDataTypeStr=boolean
  PID_max : Inport  Port=6
  Constant5 : Constant  Value=0  OutDataTypeStr=Inherit: Inherit via back propagation  SampleTime=-1
  Error : Sum  Inputs=+-
  PID : Subsystem
  Voltage_Vq : Outport  VectorParamsAs1DForOutWhenUnconnected=off
  wires:
  Current_Command/1 -> Error/1
  Current_Measured/1 -> Error/2  "current"
  Error/1 -> PID/1(Differ)  "currentControlError"
  Init_PID/1 -> PID/5(Init)
  Current_Ki/1 -> PID/3(Ki)
  Constant5/1 -> PID/4(Kd)
  PID_max/1 -> PID/6(Sat_value)
  Current_Kp/1 -> PID/2(Kp)
  PID/1(PID_Out) -> Voltage_Vq/1

== system FOC_Controller/PositionControl/Position_Control/PID ==
  Differ : Inport  OutDataTypeStr=single
  Kp : Inport  Port=2  OutDataTypeStr=single
  Ki : Inport  Port=3  OutDataTypeStr=single
  Kd : Inport  Port=4  OutDataTypeStr=single
  Init : Inport  Port=5  OutDataTypeStr=boolean
  Sat_value : Inport  Port=6  OutDataTypeStr=single
  Delay6 : Delay  DelayLength=1
  Regul : Subsystem
  Saturation : Subsystem
  Unary Minus2 : UnaryMinus
  PID_Out : Outport  VectorParamsAs1DForOutWhenUnconnected=off
  wires:
  Init/1 -> Regul/5(Init)
  Differ/1 -> Regul/1(Differ)
  Sat_value/1 -> Unary Minus2/1, Saturation/1(Max)
  Saturation/2(Enable_Sat) -> Delay6/1
  Saturation/1(Output) -> PID_Out/1
  Delay6/1 -> Regul/6(Enable_sat)
  Unary Minus2/1 -> Saturation/2(Min)
  Regul/2(PI_Out) -> Saturation/4(Input)
  Kd/1 -> Regul/4(Kd)
  Regul/1(Err_Out) -> Saturation/3(Err_in)
  Kp/1 -> Regul/2(Kp)
  Ki/1 -> Regul/3(Ki)

== system FOC_Controller/SpeedControl/Speed_Control/PID ==
  Differ : Inport  OutDataTypeStr=single
  Kp : Inport  Port=2  OutDataTypeStr=single
  Ki : Inport  Port=3  OutDataTypeStr=single
  Kd : Inport  Port=4  OutDataTypeStr=single
  Init : Inport  Port=5  OutDataTypeStr=boolean
  Sat_value : Inport  Port=6  OutDataTypeStr=single
  Delay6 : Delay  DelayLength=1
  Regul : Subsystem
  Saturation : Subsystem
  Unary Minus2 : UnaryMinus
  PID_Out : Outport  VectorParamsAs1DForOutWhenUnconnected=off
  wires:
  Init/1 -> Regul/5(Init)
  Differ/1 -> Regul/1(Differ)
  Sat_value/1 -> Unary Minus2/1, Saturation/1(Max)
  Saturation/2(Enable_Sat) -> Delay6/1
  Saturation/1(Output) -> PID_Out/1
  Delay6/1 -> Regul/6(Enable_sat)
  Unary Minus2/1 -> Saturation/2(Min)
  Regul/2(PI_Out) -> Saturation/4(Input)
  Kd/1 -> Regul/4(Kd)
  Regul/1(Err_Out) -> Saturation/3(Err_in)
  Kp/1 -> Regul/2(Kp)
  Ki/1 -> Regul/3(Ki)

== system FOC_Controller/CurrentControl/DQ_Current_Control/D_Current_Control/PID ==
  Differ : Inport  OutDataTypeStr=single
  Kp : Inport  Port=2  OutDataTypeStr=single
  Ki : Inport  Port=3  OutDataTypeStr=single
  Kd : Inport  Port=4  OutDataTypeStr=single
  Init : Inport  Port=5  OutDataTypeStr=boolean
  Sat_value : Inport  Port=6  OutDataTypeStr=single
  Delay6 : Delay  DelayLength=1
  Regul : Subsystem
  Saturation : Subsystem
  Unary Minus2 : UnaryMinus
  PID_Out : Outport  VectorParamsAs1DForOutWhenUnconnected=off
  wires:
  Init/1 -> Regul/5(Init)
  Differ/1 -> Regul/1(Differ)
  Sat_value/1 -> Unary Minus2/1, Saturation/1(Max)
  Saturation/2(Enable_Sat) -> Delay6/1
  Saturation/1(Output) -> PID_Out/1
  Delay6/1 -> Regul/6(Enable_sat)
  Unary Minus2/1 -> Saturation/2(Min)
  Regul/2(PI_Out) -> Saturation/4(Input)
  Kd/1 -> Regul/4(Kd)
  Regul/1(Err_Out) -> Saturation/3(Err_in)
  Kp/1 -> Regul/2(Kp)
  Ki/1 -> Regul/3(Ki)

== system FOC_Controller/CurrentControl/DQ_Current_Control/Q_Current_Control/PID ==
  Differ : Inport  OutDataTypeStr=single
  Kp : Inport  Port=2  OutDataTypeStr=single
  Ki : Inport  Port=3  OutDataTypeStr=single
  Kd : Inport  Port=4  OutDataTypeStr=single
  Init : Inport  Port=5  OutDataTypeStr=boolean
  Sat_value : Inport  Port=6  OutDataTypeStr=single
  Delay6 : Delay  DelayLength=1
  Regul : Subsystem
  Saturation : Subsystem
  Unary Minus2 : UnaryMinus
  PID_Out : Outport  VectorParamsAs1DForOutWhenUnconnected=off
  wires:
  Init/1 -> Regul/5(Init)
  Differ/1 -> Regul/1(Differ)
  Sat_value/1 -> Unary Minus2/1, Saturation/1(Max)
  Saturation/2(Enable_Sat) -> Delay6/1
  Saturation/1(Output) -> PID_Out/1
  Delay6/1 -> Regul/6(Enable_sat)
  Unary Minus2/1 -> Saturation/2(Min)
  Regul/2(PI_Out) -> Saturation/4(Input)
  Kd/1 -> Regul/4(Kd)
  Regul/1(Err_Out) -> Saturation/3(Err_in)
  Kp/1 -> Regul/2(Kp)
  Ki/1 -> Regul/3(Ki)

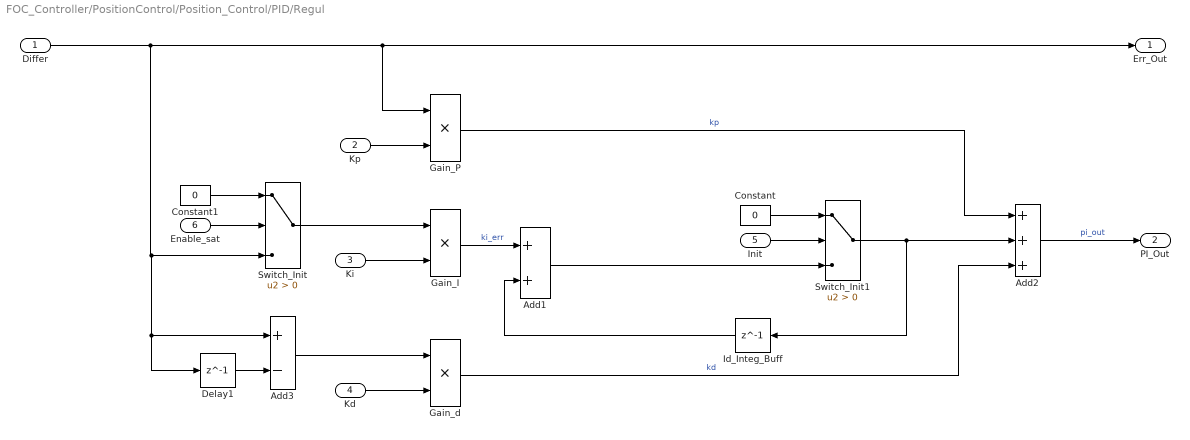
== system FOC_Controller/PositionControl/Position_Control/PID/Regul ==
  Differ : Inport
  Kp : Inport  Port=2
  Ki : Inport  Port=3
  Kd : Inport  Port=4
  Init : Inport  Port=5
  Enable_sat : Inport  Port=6
  Add1 : Sum  InputSameDT=on  SaturateOnIntegerOverflow=on  OutDataTypeStr=Inherit: Same as first input
  Add2 : Sum  Inputs=+++  InputSameDT=on  OutDataTypeStr=Inherit: Inherit via back propagation  SaturateOnIntegerOverflow=on
  Add3 : Sum  Inputs=+-  InputSameDT=on  SaturateOnIntegerOverflow=on
  Constant : Constant  Value=0  OutDataTypeStr=Inherit: Inherit via back propagation  SampleTime=-1
  Constant1 : Constant  Value=0  OutDataTypeStr=Inherit: Inherit via back propagation  SampleTime=-1
  Delay1 : Delay  DelayLength=1  InitialCondition=0
  Gain_I : Product  RndMeth=Zero  SaturateOnIntegerOverflow=on  OutDataTypeStr=Inherit: Same as first input
  Gain_P : Product  RndMeth=Zero  SaturateOnIntegerOverflow=on  OutDataTypeStr=Inherit: Same as first input
  Gain_d : Product  RndMeth=Zero  SaturateOnIntegerOverflow=on  OutDataTypeStr=Inherit: Same as first input
  Id_Integ_Buff : Delay  DelayLength=1  InitialCondition=0
  Switch_Init : Switch  Criteria=u2 > Threshold
  Switch_Init1 : Switch  Criteria=u2 > Threshold  OutDataTypeStr=Inherit: Inherit via back propagation  InputSameDT=on
  Err_Out : Outport  InitialOutput=0  VectorParamsAs1DForOutWhenUnconnected=off
  PI_Out : Outport  Port=2  InitialOutput=0  VectorParamsAs1DForOutWhenUnconnected=off
  wires:
  Kd/1 -> Gain_d/2
  Gain_d/1 -> Add2/3  "kd"
  Add3/1 -> Gain_d/1
  Delay1/1 -> Add3/2
  Constant/1 -> Switch_Init1/1
  Add1/1 -> Switch_Init1/3
  Enable_sat/1 -> Switch_Init/2
  Constant1/1 -> Switch_Init/1
  Init/1 -> Switch_Init1/2
  Gain_I/1 -> Add1/1  "ki_err"
  Gain_P/1 -> Add2/1  "kp"
  Differ/1 -> Err_Out/1, Gain_P/1, Switch_Init/3, Add3/1, Delay1/1
  Add2/1 -> PI_Out/1  "pi_out"
  Switch_Init1/1 -> Id_Integ_Buff/1, Add2/2
  Id_Integ_Buff/1 -> Add1/2
  Kp/1 -> Gain_P/2
  Ki/1 -> Gain_I/2
  Switch_Init/1 -> Gain_I/1

== system FOC_Controller/PositionControl/Position_Control/PID/Saturation ==
  note: %大于最大值时，偏差仍为正，
      | 或小于最小值时，偏差仍为负，
      | 此时积分饱和限值%
  note: range[-AbsVmax~AbsVmax]
  Max : Inport
  Min : Inport  Port=2
  Err_in : Inport  Port=3
  Input : Inport  Port=4
  CompZero1 : simulink/Logic and Bit Operations/Compare To Zero  relop=<  OutDataTypeStr=boolean
  CompZero2 : simulink/Logic and Bit Operations/Compare To Zero  relop=>  OutDataTypeStr=boolean
  LogicalOperator1 : Logic  OutDataTypeStr=boolean
  LogicalOperator2 : Logic  OutDataTypeStr=boolean
  LogicalOperator3 : Logic  Operator=OR  OutDataTypeStr=boolean
  Sat : Subsystem
  Output : Outport  InitialOutput=0  VectorParamsAs1DForOutWhenUnconnected=off
  Enable_Sat : Outport  Port=2  InitialOutput=0  VectorParamsAs1DForOutWhenUnconnected=off
  wires:
  Max/1 -> Sat/1(Val_Max)
  Input/1 -> Sat/3(Val)
  Min/1 -> Sat/2(Val_Min)
  Sat/1(Val_Out) -> Output/1
  Sat/2(SatMax) -> LogicalOperator1/1
  Sat/3(SatMin) -> LogicalOperator2/1
  Err_in/1 -> CompZero1/1, CompZero2/1
  CompZero2/1 -> LogicalOperator1/2
  CompZero1/1 -> LogicalOperator2/2
  LogicalOperator1/1 -> LogicalOperator3/1
  LogicalOperator2/1 -> LogicalOperator3/2
  LogicalOperator3/1 -> Enable_Sat/1

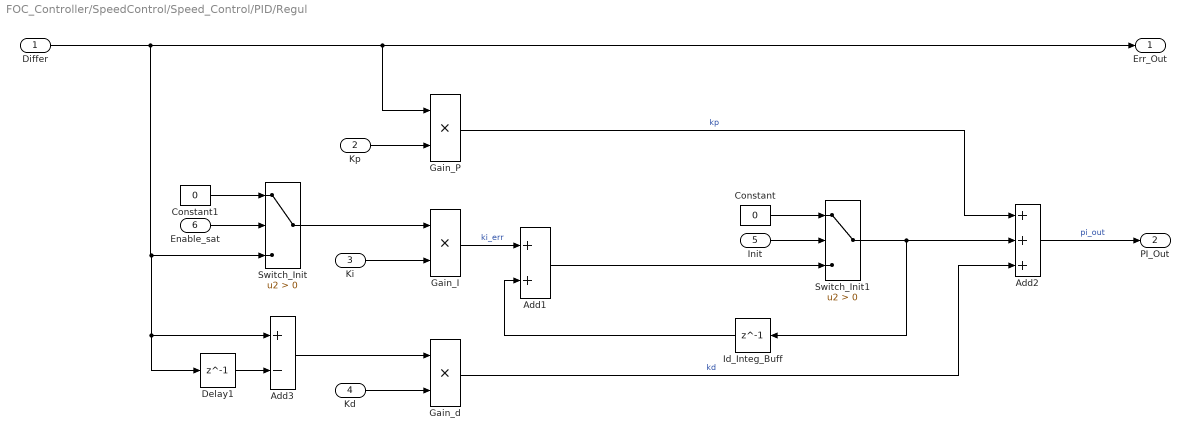
== system FOC_Controller/SpeedControl/Speed_Control/PID/Regul ==
  Differ : Inport
  Kp : Inport  Port=2
  Ki : Inport  Port=3
  Kd : Inport  Port=4
  Init : Inport  Port=5
  Enable_sat : Inport  Port=6
  Add1 : Sum  InputSameDT=on  SaturateOnIntegerOverflow=on  OutDataTypeStr=Inherit: Same as first input
  Add2 : Sum  Inputs=+++  InputSameDT=on  OutDataTypeStr=Inherit: Inherit via back propagation  SaturateOnIntegerOverflow=on
  Add3 : Sum  Inputs=+-  InputSameDT=on  SaturateOnIntegerOverflow=on
  Constant : Constant  Value=0  OutDataTypeStr=Inherit: Inherit via back propagation  SampleTime=-1
  Constant1 : Constant  Value=0  OutDataTypeStr=Inherit: Inherit via back propagation  SampleTime=-1
  Delay1 : Delay  DelayLength=1  InitialCondition=0
  Gain_I : Product  RndMeth=Zero  SaturateOnIntegerOverflow=on  OutDataTypeStr=Inherit: Same as first input
  Gain_P : Product  RndMeth=Zero  SaturateOnIntegerOverflow=on  OutDataTypeStr=Inherit: Same as first input
  Gain_d : Product  RndMeth=Zero  SaturateOnIntegerOverflow=on  OutDataTypeStr=Inherit: Same as first input
  Id_Integ_Buff : Delay  DelayLength=1  InitialCondition=0
  Switch_Init : Switch  Criteria=u2 > Threshold
  Switch_Init1 : Switch  Criteria=u2 > Threshold  OutDataTypeStr=Inherit: Inherit via back propagation  InputSameDT=on
  Err_Out : Outport  InitialOutput=0  VectorParamsAs1DForOutWhenUnconnected=off
  PI_Out : Outport  Port=2  InitialOutput=0  VectorParamsAs1DForOutWhenUnconnected=off
  wires:
  Kd/1 -> Gain_d/2
  Gain_d/1 -> Add2/3  "kd"
  Add3/1 -> Gain_d/1
  Delay1/1 -> Add3/2
  Constant/1 -> Switch_Init1/1
  Add1/1 -> Switch_Init1/3
  Enable_sat/1 -> Switch_Init/2
  Constant1/1 -> Switch_Init/1
  Init/1 -> Switch_Init1/2
  Gain_I/1 -> Add1/1  "ki_err"
  Gain_P/1 -> Add2/1  "kp"
  Differ/1 -> Err_Out/1, Gain_P/1, Switch_Init/3, Add3/1, Delay1/1
  Add2/1 -> PI_Out/1  "pi_out"
  Switch_Init1/1 -> Id_Integ_Buff/1, Add2/2
  Id_Integ_Buff/1 -> Add1/2
  Kp/1 -> Gain_P/2
  Ki/1 -> Gain_I/2
  Switch_Init/1 -> Gain_I/1

== system FOC_Controller/SpeedControl/Speed_Control/PID/Saturation ==
  note: %大于最大值时，偏差仍为正，
      | 或小于最小值时，偏差仍为负，
      | 此时积分饱和限值%
  note: range[-AbsVmax~AbsVmax]
  Max : Inport
  Min : Inport  Port=2
  Err_in : Inport  Port=3
  Input : Inport  Port=4
  CompZero1 : simulink/Logic and Bit Operations/Compare To Zero  relop=<  OutDataTypeStr=boolean
  CompZero2 : simulink/Logic and Bit Operations/Compare To Zero  relop=>  OutDataTypeStr=boolean
  LogicalOperator1 : Logic  OutDataTypeStr=boolean
  LogicalOperator2 : Logic  OutDataTypeStr=boolean
  LogicalOperator3 : Logic  Operator=OR  OutDataTypeStr=boolean
  Sat : Subsystem
  Output : Outport  InitialOutput=0  VectorParamsAs1DForOutWhenUnconnected=off
  Enable_Sat : Outport  Port=2  InitialOutput=0  VectorParamsAs1DForOutWhenUnconnected=off
  wires:
  Max/1 -> Sat/1(Val_Max)
  Input/1 -> Sat/3(Val)
  Min/1 -> Sat/2(Val_Min)
  Sat/1(Val_Out) -> Output/1
  Sat/2(SatMax) -> LogicalOperator1/1
  Sat/3(SatMin) -> LogicalOperator2/1
  Err_in/1 -> CompZero1/1, CompZero2/1
  CompZero2/1 -> LogicalOperator1/2
  CompZero1/1 -> LogicalOperator2/2
  LogicalOperator1/1 -> LogicalOperator3/1
  LogicalOperator2/1 -> LogicalOperator3/2
  LogicalOperator3/1 -> Enable_Sat/1

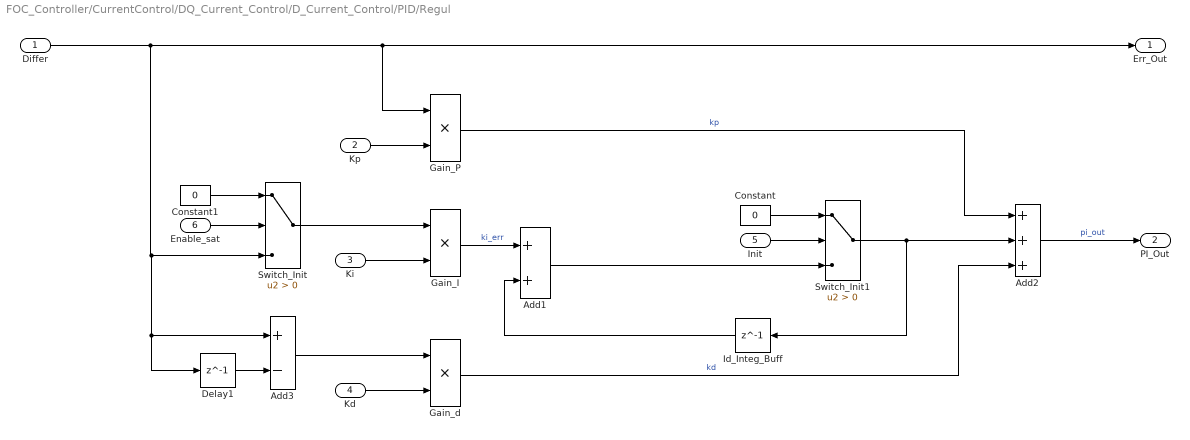
== system FOC_Controller/CurrentControl/DQ_Current_Control/D_Current_Control/PID/Regul ==
  Differ : Inport
  Kp : Inport  Port=2
  Ki : Inport  Port=3
  Kd : Inport  Port=4
  Init : Inport  Port=5
  Enable_sat : Inport  Port=6
  Add1 : Sum  InputSameDT=on  SaturateOnIntegerOverflow=on  OutDataTypeStr=Inherit: Same as first input
  Add2 : Sum  Inputs=+++  InputSameDT=on  OutDataTypeStr=Inherit: Inherit via back propagation  SaturateOnIntegerOverflow=on
  Add3 : Sum  Inputs=+-  InputSameDT=on  SaturateOnIntegerOverflow=on
  Constant : Constant  Value=0  OutDataTypeStr=Inherit: Inherit via back propagation  SampleTime=-1
  Constant1 : Constant  Value=0  OutDataTypeStr=Inherit: Inherit via back propagation  SampleTime=-1
  Delay1 : Delay  DelayLength=1  InitialCondition=0
  Gain_I : Product  RndMeth=Zero  SaturateOnIntegerOverflow=on  OutDataTypeStr=Inherit: Same as first input
  Gain_P : Product  RndMeth=Zero  SaturateOnIntegerOverflow=on  OutDataTypeStr=Inherit: Same as first input
  Gain_d : Product  RndMeth=Zero  SaturateOnIntegerOverflow=on  OutDataTypeStr=Inherit: Same as first input
  Id_Integ_Buff : Delay  DelayLength=1  InitialCondition=0
  Switch_Init : Switch  Criteria=u2 > Threshold
  Switch_Init1 : Switch  Criteria=u2 > Threshold  OutDataTypeStr=Inherit: Inherit via back propagation  InputSameDT=on
  Err_Out : Outport  InitialOutput=0  VectorParamsAs1DForOutWhenUnconnected=off
  PI_Out : Outport  Port=2  InitialOutput=0  VectorParamsAs1DForOutWhenUnconnected=off
  wires:
  Kd/1 -> Gain_d/2
  Gain_d/1 -> Add2/3  "kd"
  Add3/1 -> Gain_d/1
  Delay1/1 -> Add3/2
  Constant/1 -> Switch_Init1/1
  Add1/1 -> Switch_Init1/3
  Enable_sat/1 -> Switch_Init/2
  Constant1/1 -> Switch_Init/1
  Init/1 -> Switch_Init1/2
  Gain_I/1 -> Add1/1  "ki_err"
  Gain_P/1 -> Add2/1  "kp"
  Differ/1 -> Err_Out/1, Gain_P/1, Switch_Init/3, Add3/1, Delay1/1
  Add2/1 -> PI_Out/1  "pi_out"
  Switch_Init1/1 -> Id_Integ_Buff/1, Add2/2
  Id_Integ_Buff/1 -> Add1/2
  Kp/1 -> Gain_P/2
  Ki/1 -> Gain_I/2
  Switch_Init/1 -> Gain_I/1

== system FOC_Controller/CurrentControl/DQ_Current_Control/D_Current_Control/PID/Saturation ==
  note: %大于最大值时，偏差仍为正，
      | 或小于最小值时，偏差仍为负，
      | 此时积分饱和限值%
  note: range[-AbsVmax~AbsVmax]
  Max : Inport
  Min : Inport  Port=2
  Err_in : Inport  Port=3
  Input : Inport  Port=4
  CompZero1 : simulink/Logic and Bit Operations/Compare To Zero  relop=<  OutDataTypeStr=boolean
  CompZero2 : simulink/Logic and Bit Operations/Compare To Zero  relop=>  OutDataTypeStr=boolean
  LogicalOperator1 : Logic  OutDataTypeStr=boolean
  LogicalOperator2 : Logic  OutDataTypeStr=boolean
  LogicalOperator3 : Logic  Operator=OR  OutDataTypeStr=boolean
  Sat : Subsystem
  Output : Outport  InitialOutput=0  VectorParamsAs1DForOutWhenUnconnected=off
  Enable_Sat : Outport  Port=2  InitialOutput=0  VectorParamsAs1DForOutWhenUnconnected=off
  wires:
  Max/1 -> Sat/1(Val_Max)
  Input/1 -> Sat/3(Val)
  Min/1 -> Sat/2(Val_Min)
  Sat/1(Val_Out) -> Output/1
  Sat/2(SatMax) -> LogicalOperator1/1
  Sat/3(SatMin) -> LogicalOperator2/1
  Err_in/1 -> CompZero1/1, CompZero2/1
  CompZero2/1 -> LogicalOperator1/2
  CompZero1/1 -> LogicalOperator2/2
  LogicalOperator1/1 -> LogicalOperator3/1
  LogicalOperator2/1 -> LogicalOperator3/2
  LogicalOperator3/1 -> Enable_Sat/1
